simulink model "flyback_70khz"  (R2021b)
settings: Solver=VariableStepAuto  StartTime=0.0  StopTime=0.05  RelTol=1e-3
libraries: spsCurrentMeasurementLib x3, spsSeriesRLCBranchLib x2, spsMultimeterLib x2, spsRMSLib x2, spsDiodeLib x1, spsLinearTransformerLib x1, spsMosfetLib x1, spsDCVoltageSourceLib x1, spsVoltageMeasurementLib x1, spspowerguiLib x1
settings Model: Creator=pc  LastModifiedBy=pc

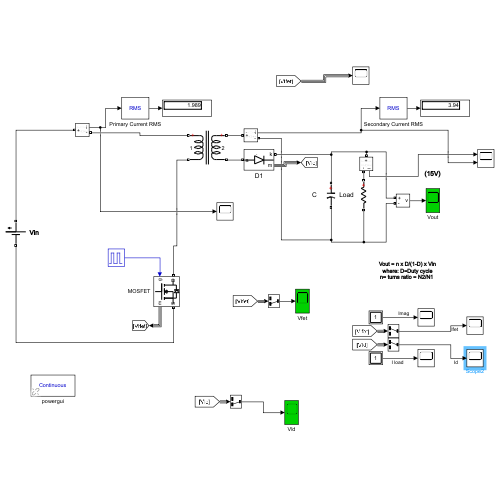
[thumbnail: Simulink's stored preview of the top-level diagram]
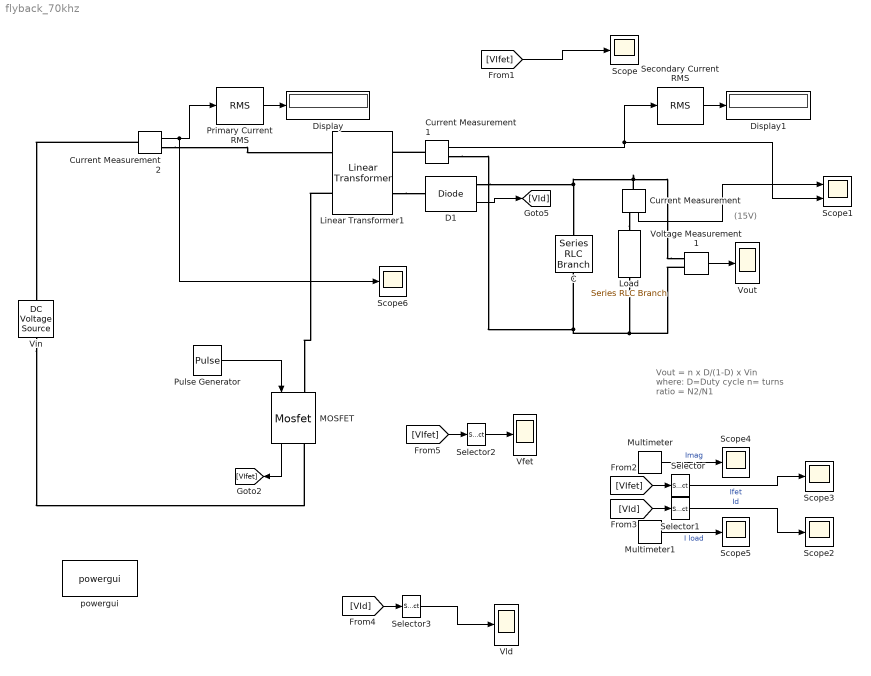
== system flyback_70khz ==
  note: (15V)
  note: Vout = n x D/(1-D) x Vin
      | where: D=Duty cycle
      | n= turns ratio = N2/N1
  C : spsSeriesRLCBranchLib/Series RLC Branch  LConnTagsString=__new0  RConnTagsString=__new0  BranchType=C  Resistance=1e-4  Inductance=200e-6  SetiL0=off  InitialCurrent=0  Capacitance=50e-6  Setx0=off  InitialVoltage=0  Measurements=None
  Current Measurement : spsCurrentMeasurementLib/Current Measurement  PhasorSimulation=off  OutputType=Complex  PSBequivalent=0
  Current Measurement1 : spsCurrentMeasurementLib/Current Measurement  PhasorSimulation=off  OutputType=Complex  PSBequivalent=0
  Current Measurement2 : spsCurrentMeasurementLib/Current Measurement  PhasorSimulation=off  OutputType=Complex  PSBequivalent=0
  D1 : spsDiodeLib/Diode  Ron=1e-3  Lon=0  Vf=0  IC=0  UseSnubber=off  Rs=inf  Cs=0  Measurements=on
  Display : Display
  Display1 : Display
  Linear Transformer1 : spsLinearTransformerLib/Linear Transformer  UNITS=SI  NominalPower=[45 7e4 ]  winding1=[20 0 0]  winding2=[15 0 0]  ThreeWindings=off  winding3=[3.15e+05 0.7938 1.6845e-05]  RmLm=[inf 46e-6]  Measurements=Magnetization current  DataType=on
  Load : spsSeriesRLCBranchLib/Series RLC Branch  LConnTagsString=__new0  RConnTagsString=__new0  BranchType=R  Resistance=5  Inductance=200e-6  SetiL0=off  InitialCurrent=0  Capacitance=400e-6  Setx0=off  InitialVoltage=0  Measurements=Branch current
  MOSFET : spsMosfetLib/Mosfet  Ron=0  Lon=0  Rd=0  Vfd=0  IC=0  Rs=1e6  Cs=inf  Measurements=on
  Multimeter : spsMultimeterLib/Multimeter  PhasorSimulation=off  OutputType=Complex  sel=3  L=4  Gain=1  yselected={'Imag: Linear Transformer1'};  PSBOutputType=1  PSBequivalent=0  AxesSetting=[0,0.1,-100,100]  Display=0  SavedBlockNames=-11
  Multimeter1 : spsMultimeterLib/Multimeter  PhasorSimulation=off  OutputType=Complex  sel=1  L=4  Gain=1  yselected={'Ib: Load'};  PSBOutputType=1  PSBequivalent=0  AxesSetting=[0,0.1,-100,100]  Display=0  SavedBlockNames=-11
  Primary Current RMS : spsRMSLib/RMS  TrueRMS=on  Freq=60  RMSInit=120  Ts=0
  Pulse Generator : DiscretePulseGenerator  PulseType=Time based  Period=1/70e3  PulseWidth=29.36
  Scope{,2..6} (6 alike) : Scope
  Scope1 : Scope  NumInputPorts=2
  Secondary Current RMS : spsRMSLib/RMS  TrueRMS=on  Freq=60  RMSInit=120  Ts=0
  Selector : Selector  InputPortWidth=2  IndexOptions=Index vector (dialog)  Indices=1  OutputSizes=1
  Selector1 : Selector  InputPortWidth=2  IndexOptions=Index vector (dialog)  Indices=1  OutputSizes=1
  Selector2 : Selector  InputPortWidth=2  IndexOptions=Index vector (dialog)  Indices=2  OutputSizes=1
  Selector3 : Selector  InputPortWidth=2  IndexOptions=Index vector (dialog)  Indices=2  OutputSizes=1
  Vfet : Scope
  Vin : spsDCVoltageSourceLib/DC Voltage Source  Amplitude=48  Measurements=None
  Vld : Scope
  Voltage Measurement1 : spsVoltageMeasurementLib/Voltage Measurement  PhasorSimulation=off  OutputType=Complex  PSBequivalent=0
  Vout : Scope
  powergui : spspowerguiLib/powergui  Priority=1  SimulationMode=Continuous  SampleTime=50e-6  frequency=60  Iterations=50  frequencyindice=0  Pbase=100e6  ErrMax=1e-4  UnitsV=kV  UnitsW=MW  buscounter=0  FunctionMessages=off  echomessages=off  EnableUseOfTLC=off  CurrentSourceSwitches=off  DisableSnubberDevices=off  DisableRonSwitches=off  DisableVfSwitches=off  DisplayEquations=off  AutomaticDiscreteSolvers=off  SolverType=Tustin/Backward Euler (TBE)  Interpol=off  ExternalGateDelay=off  methode=off  Ts=100  x0status=blocks  SPID=on  SwTol=0  HookPort=off  NonlinearTolerance=1e-4  nMaxIteration=100  ContinueOnMaxIteration=off  RestoreLinks=warning  ResistiveCurrentMeasurement=off  Frange=[0:2:500]  Ylog=off  Xlog=on  ShowGrid=off  save=off  variable=ZData  structure=0  ZoomFFT=off  StartTime=0.0  cycles=1  DisplayStyle=1  fundamental=60  FreqAxis=off  MaxFrequency=1000  frequencyindicesteady=1  RmsSteady=1  display=off
  wires:
  Selector1/1 -> Scope2/1  "Id"
  Current Measurement2/1 -> Scope6/1, Primary Current RMS/1
  Current Measurement1/1 -> Secondary Current RMS/1, Scope1/2
  [VIfet] -> Scope/1
  [VId] -> Selector3/1
  Secondary Current RMS/1 -> Display1/1
  [VIfet] -> Selector/1
  [VIfet] -> Selector2/1
  Multimeter1/1 -> Scope5/1  "I load"
  Current Measurement/1 -> Scope1/1
  Multimeter/1 -> Scope4/1  "Imag"
  Selector2/1 -> Vfet/1
  Selector3/1 -> Vld/1
  MOSFET/1 -> [VIfet]
  Primary Current RMS/1 -> Display/1
  Voltage Measurement1/1 -> Vout/1
  Pulse Generator/1 -> MOSFET/1
  [VId] -> Selector1/1
  Selector/1 -> Scope3/1  "Ifet"
  D1/1 -> [VId]
  connections:
  C/RConn1 -- Current Measurement1/RConn1 -- Load/RConn1 -- Voltage Measurement1/LConn2
  Voltage Measurement1/LConn1 -- D1/RConn1 -- C/LConn1 -- Current Measurement/LConn1
  Vin/LConn1 -- MOSFET/RConn1
  Current Measurement/RConn1 -- Load/LConn1
  Current Measurement1/LConn1 -- Linear Transformer1/RConn1
  Current Measurement2/LConn1 -- Vin/RConn1
  Current Measurement2/RConn1 -- Linear Transformer1/LConn1
  Linear Transformer1/RConn2 -- D1/LConn1
  Linear Transformer1/LConn2 -- MOSFET/LConn1
